simulink model "sistema1"  (R2026a)
settings: Solver=VariableStepAuto
libraries: simulink x1, slpidlib x1
settings DataIOCC: TimeSaveName=t
settings DebuggingCC: ArtificialAlgebraicLoopMsg=none  MaxConsecutiveZCsMsg=none

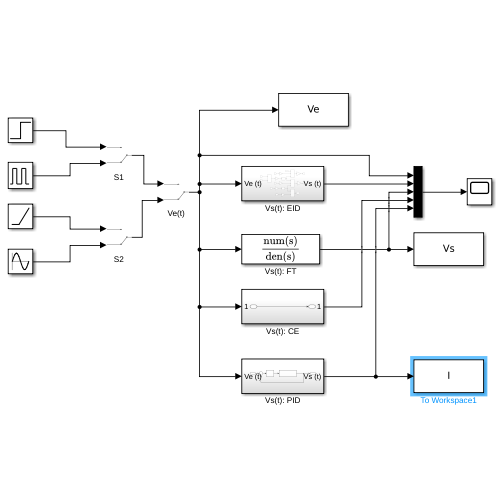
[thumbnail: Simulink's stored preview of the top-level diagram]
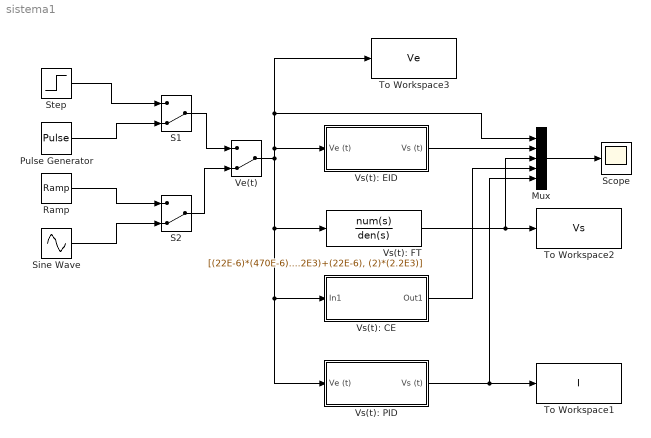
== system sistema1 ==
  Mux : Mux  Inputs=5
  Pulse Generator : DiscretePulseGenerator  PulseType=Time based  Period=10  PulseWidth=10  PhaseDelay=1
  Ramp : simulink/Sources/Ramp  slope=1/10  start=0  InitialOutput=0
  S1 : ManualSwitch  CurrentSetting=0
  S2 : ManualSwitch  CurrentSetting=0
  Scope : Scope
      settings: ActiveDisplayYMinimum=-0.63510679787637314  ActiveDisplayYMaximum=0.96024515524862819
  Sine Wave : Sin  Frequency=pi/2  SampleTime=0
  Step : Step  Time=0  SampleTime=0
  To Workspace1 : ToWorkspace  VariableName=I  SampleTime=-1
  To Workspace2 : ToWorkspace  VariableName=Vs  SampleTime=-1
  To Workspace3 : ToWorkspace  VariableName=Ve  SampleTime=-1
  Ve(t) : ManualSwitch  CurrentSetting=0
  Vs(t): CE : Subsystem
  Vs(t): EID : Subsystem
  Vs(t): FT : TransferFcn  Numerator=[(22E-6)*(470E-6)*(2.2E3), (2.2E3)*(470E-6)*(2.2E3)+(22E-6), 2.2E3]  Denominator=[(3)*(22E-6)*(470E-6)*(2.2E3), (5)*(2.2E3)*(470E-6)*(2.2E3)+(22E-6), (2)*(2.2E3)]
  Vs(t): PID : Subsystem
  wires:
  Step/1 -> S1/1
  Pulse Generator/1 -> S1/2
  Ramp/1 -> S2/1
  Sine Wave/1 -> S2/2
  S1/1 -> Ve(t)/1
  S2/1 -> Ve(t)/2
  Ve(t)/1 -> To Workspace3/1, Mux/1, Vs(t): EID/1(Ve (t)), Vs(t): CE/1(In1), Vs(t): PID/1(Ve (t)), Vs(t): FT/1
  Mux/1 -> Scope/1
  Vs(t): FT/1 -> To Workspace2/1, Mux/3
  Vs(t): PID/1(Vs (t)) -> Mux/5, To Workspace1/1
  Vs(t): EID/1(Vs (t)) -> Mux/2
  Vs(t): CE/1(Out1) -> Mux/4

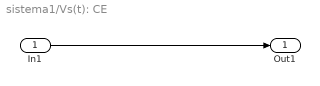
== system sistema1/Vs(t): CE ==
  In1 : Inport
  Out1 : Outport
  wires:
  In1/1 -> Out1/1

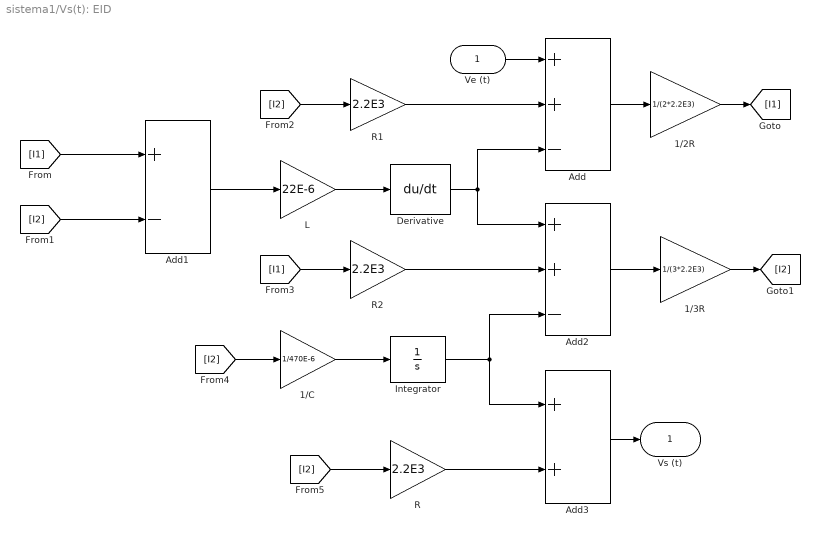
== system sistema1/Vs(t): EID ==
  Ve (t) : Inport
  1/2R : Gain  Gain=1/(2*2.2E3)
  1/3R : Gain  Gain=1/(3*2.2E3)
  1/C : Gain  Gain=1/470E-6
  Add : Sum  Inputs=++-
  Add1 : Sum  Inputs=+-
  Add2 : Sum  Inputs=++-
  Add3 : Sum
  Derivative : Derivative
  Integrator : Integrator
  L : Gain  Gain=22E-6
  R : Gain  Gain=2.2E3
  R1 : Gain  Gain=2.2E3
  R2 : Gain  Gain=2.2E3
  Vs (t) : Outport
  wires:
  Ve (t)/1 -> Add/1
  R1/1 -> Add/2
  L/1 -> Derivative/1
  Derivative/1 -> Add/3, Add2/1
  Add1/1 -> L/1
  [I1] -> Add1/1
  [I2] -> Add1/2
  [I2] -> R1/1
  Add/1 -> 1/2R/1
  1/2R/1 -> [I1]
  1/C/1 -> Integrator/1
  Integrator/1 -> Add3/1, Add2/3
  R2/1 -> Add2/2
  R/1 -> Add3/2
  1/3R/1 -> [I2]
  Add2/1 -> 1/3R/1
  Add3/1 -> Vs (t)/1
  [I1] -> R2/1
  [I2] -> 1/C/1
  [I2] -> R/1

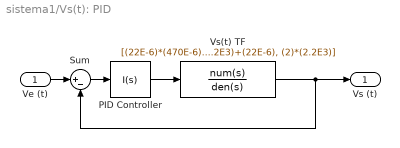
== system sistema1/Vs(t): PID ==
  Ve (t) : Inport
  PID Controller : slpidlib/PID Controller  Controller=I  Form=Parallel  TimeDomain=Continuous-time  UseExternalTs=off  SampleTime=-1  IntegratorMethod=Forward Euler  FilterMethod=Forward Euler  ControllerParametersSource=internal  P=239.6613  I=171.1222  UseKiTs=off  D=0.39134  UseExternalDerivativeSource=off  N=502.9743  UseFilter=on  TunerSelectOption=Transfer Function Based (PID Tuner App)  InitialConditionSource=internal  InitialConditionForIntegrator=0  InitialConditionForFilter=0  DifferentiatorICPrevScaledInput=0  ExternalReset=none  TrackingMode=off  Kt=1  LimitOutput=off  SatLimitsSource=internal  UpperSaturationLimit=inf  LowerSaturationLimit=-inf  LinearizeAsGain=on  AntiWindupMode=none  Kb=1  LimitIntegrator=off  UpperIntegratorSaturationLimit=inf  LowerIntegratorSaturationLimit=-inf  POutMin=[]  POutMax=[]  IOutMin=[]  IOutMax=[]  DOutMin=[]  DOutMax=[]  NOutMin=[]  NOutMax=[]  SumOutMin=[]  SumOutMax=[]  SaturationOutMin=[]  SaturationOutMax=[]  PParamMin=[]  PParamMax=[]  IParamMin=[]  IParamMax=[]  DParamMin=[]  DParamMax=[]  NParamMin=[]  NParamMax=[]  KbParamMin=[]  KbParamMax=[]  KtParamMin=[]  KtParamMax=[]  KbOutMin=[]  KbOutMax=[]  KtOutMin=[]  KtOutMax=[]  IntegratorOutMin=[]  IntegratorOutMax=[]  FilterOutMin=[]  FilterOutMax=[]  SumI1OutMin=[]  SumI1OutMax=[]  SumI2OutMin=[]  SumI2OutMax=[]  SumI3OutMin=[]  SumI3OutMax=[]  SumI4OutMin=[]  SumI4OutMax=[]  SumDOutMin=[]  SumDOutMax=[]  DifferentiatorOutMin=[]  DifferentiatorOutMax=[]  FilterDiffOutCoefMin=[]  FilterDiffOutCoefMax=[]  ReciprocalOutMin=[]  ReciprocalOutMax=[]  SumDenOutMin=[]  SumDenOutMax=[]  SumNumOutMin=[]  SumNumOutMax=[]  DivideOutMin=[]  DivideOutMax=[]  UdiffTsProdOutMin=[]  UdiffTsProdOutMax=[]  NTsProdOutMin=[]  NTsProdOutMax=[]  UintegralTsProdOutMin=[]  UintegralTsProdOutMax=[]  UngainTsProdOutMin=[]  UngainTsProdOutMax=[]  ClampingZeroOutDataTypeStr=Inherit: Inherit via back propagation  ClampingZeroOutMin=[]  ClampingZeroOutMax=[]  FilterDenConstantOutDataTypeStr=Inherit: Inherit via back propagation  FilterDenConstantOutMin=[]  FilterDenConstantOutMax=[]  PCopyOutDataTypeStr=Inherit: Inherit via back propagation  PCopyOutMin=[]  PCopyOutMax=[]  NCopyOutDataTypeStr=Inherit: Inherit via back propagation  NCopyOutMin=[]  NCopyOutMax=[]  IntegratorContinuousStateAttributes=''  IntegratorStateMustResolveToSignalObject=off  IntegratorRTWStateStorageClass=Auto  FilterContinuousStateAttributes=''  FilterStateMustResolveToSignalObject=off  FilterRTWStateStorageClass=Auto  ParallelPVariant=Disabled  IdealPVariant=Disabled  IVariant=InternalParameters  DVariant=Disabled  IntegratorVariant=Continuous  SatVariant=Disabled  AWVariant=Passthrough  PCopyVariant=Disabled  TRVariant=Disabled  FdbkBlocksVariant=Forward  IdealPFdbkVariant=Disabled  SatFdbkVariant=Disabled  DerivativeFilterVariant=Disabled  NVariant=Disabled  NCopyVariant=Disabled_SignalSpec  FilterICVariant=Disabled  IntegratorICVariant=InternalICs  ExternalResetVariant=Disabled  TRSumVariant=Passthrough  SumFdbkVariant=Disabled  SumVariant=Passthrough_I  TsampFilterVariant=InternalTs  TsampNgainVariant=Passthrough  TsampIntegralVariant=Disabled_SignalSpec  ExternalSaturationOutDataTypeStr=Inherit: Same as second input  DerivativeSourceVariant=Disabled  PreIntVariant=InternalPreInt
  Sum : Sum  Inputs=|+-
  Vs(t) TF : TransferFcn  Numerator=[(22E-6)*(470E-6)*(2.2E3), (2.2E3)*(470E-6)*(2.2E3)+(22E-6), 2.2E3]  Denominator=[(3)*(22E-6)*(470E-6)*(2.2E3), (5)*(2.2E3)*(470E-6)*(2.2E3)+(22E-6), (2)*(2.2E3)]
  Vs (t) : Outport
  wires:
  Sum/1 -> PID Controller/1
  PID Controller/1 -> Vs(t) TF/1
  Ve (t)/1 -> Sum/1
  Vs(t) TF/1 -> Vs (t)/1, Sum/2
